simulink model "DrishtiSetu_Screening"  (R2026a)
settings: Solver=FixedStepDiscrete  StopTime=0  FixedStep=1
undefined symbols (not defined in the file or in its folder): sim_adherence, sim_camp_days, sim_devices, sim_dm_prev, sim_pop
settings Model: Creator=itsam  LastModifiedBy=itsam

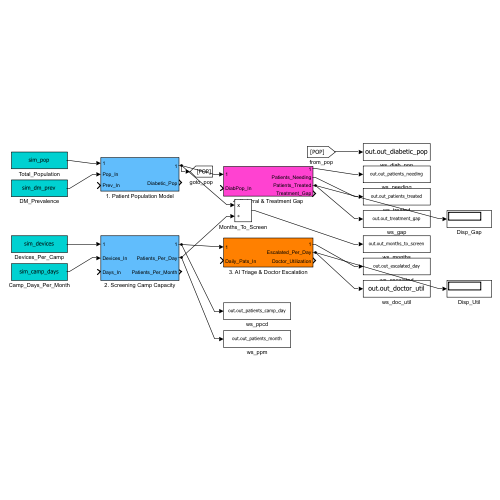
[thumbnail: Simulink's stored preview of the top-level diagram]
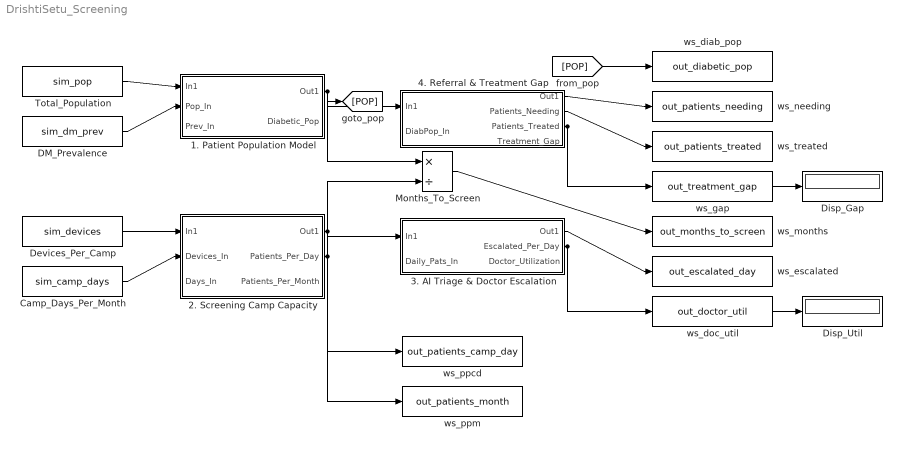
== system DrishtiSetu_Screening ==
  1. Patient Population Model : Subsystem
  2. Screening Camp Capacity : Subsystem
  3. AI Triage & Doctor Escalation : Subsystem
  4. Referral & Treatment Gap : Subsystem
  Camp_Days_Per_Month : Constant  Value=sim_camp_days
  DM_Prevalence : Constant  Value=sim_dm_prev
  Devices_Per_Camp : Constant  Value=sim_devices
  Disp_Gap : Display
  Disp_Util : Display
  Months_To_Screen : Product  Inputs=*/
  Total_Population : Constant  Value=sim_pop
  ws_diab_pop : ToWorkspace  VariableName=out_diabetic_pop  SaveFormat=Timeseries  SampleTime=-1
  ws_doc_util : ToWorkspace  VariableName=out_doctor_util  SaveFormat=Timeseries  SampleTime=-1
  ws_escalated : ToWorkspace  VariableName=out_escalated_day  SaveFormat=Timeseries  SampleTime=-1
  ws_gap : ToWorkspace  VariableName=out_treatment_gap  SaveFormat=Timeseries  SampleTime=-1
  ws_months : ToWorkspace  VariableName=out_months_to_screen  SaveFormat=Timeseries  SampleTime=-1
  ws_needing : ToWorkspace  VariableName=out_patients_needing  SaveFormat=Timeseries  SampleTime=-1
  ws_ppcd : ToWorkspace  VariableName=out_patients_camp_day  SaveFormat=Timeseries  SampleTime=-1
  ws_ppm : ToWorkspace  VariableName=out_patients_month  SaveFormat=Timeseries  SampleTime=-1
  ws_treated : ToWorkspace  VariableName=out_patients_treated  SaveFormat=Timeseries  SampleTime=-1
  wires:
  Total_Population/1 -> 1. Patient Population Model/1(In1)
  DM_Prevalence/1 -> 1. Patient Population Model/2(Pop_In)
  Devices_Per_Camp/1 -> 2. Screening Camp Capacity/1(In1)
  Camp_Days_Per_Month/1 -> 2. Screening Camp Capacity/2(Devices_In)
  2. Screening Camp Capacity/1(Out1) -> 3. AI Triage & Doctor Escalation/1(In1), ws_ppcd/1
  1. Patient Population Model/1(Out1) -> 4. Referral & Treatment Gap/1(In1), Months_To_Screen/1, [POP]
  2. Screening Camp Capacity/2(Patients_Per_Day) -> Months_To_Screen/2, ws_ppm/1
  [POP] -> ws_diab_pop/1
  4. Referral & Treatment Gap/1(Out1) -> ws_needing/1
  4. Referral & Treatment Gap/2(Patients_Needing) -> ws_treated/1
  4. Referral & Treatment Gap/3(Patients_Treated) -> ws_gap/1, Disp_Gap/1
  Months_To_Screen/1 -> ws_months/1
  3. AI Triage & Doctor Escalation/1(Out1) -> ws_escalated/1
  3. AI Triage & Doctor Escalation/2(Escalated_Per_Day) -> ws_doc_util/1, Disp_Util/1

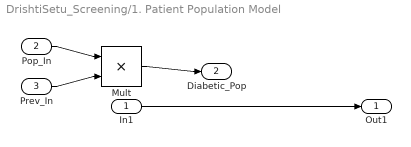
== system DrishtiSetu_Screening/1. Patient Population Model ==
  In1 : Inport
  Pop_In : Inport  Port=2
  Prev_In : Inport  Port=3
  Mult : Product
  Out1 : Outport
  Diabetic_Pop : Outport  Port=2
  wires:
  In1/1 -> Out1/1
  Pop_In/1 -> Mult/1
  Prev_In/1 -> Mult/2
  Mult/1 -> Diabetic_Pop/1

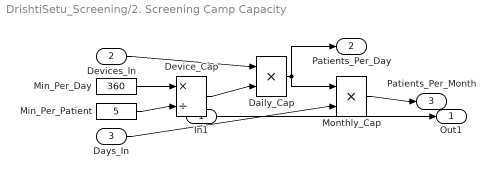
== system DrishtiSetu_Screening/2. Screening Camp Capacity ==
  In1 : Inport
  Devices_In : Inport  Port=2
  Days_In : Inport  Port=3
  Daily_Cap : Product
  Device_Cap : Product  Inputs=*/
  Min_Per_Day : Constant  Value=360
  Min_Per_Patient : Constant  Value=5
  Monthly_Cap : Product
  Out1 : Outport
  Patients_Per_Day : Outport  Port=2
  Patients_Per_Month : Outport  Port=3
  wires:
  In1/1 -> Out1/1
  Min_Per_Day/1 -> Device_Cap/1
  Min_Per_Patient/1 -> Device_Cap/2
  Devices_In/1 -> Daily_Cap/1
  Device_Cap/1 -> Daily_Cap/2
  Daily_Cap/1 -> Monthly_Cap/1, Patients_Per_Day/1
  Days_In/1 -> Monthly_Cap/2
  Monthly_Cap/1 -> Patients_Per_Month/1

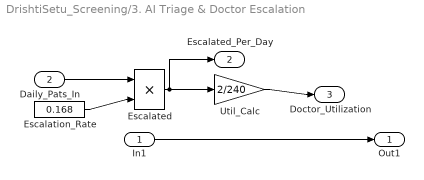
== system DrishtiSetu_Screening/3. AI Triage & Doctor Escalation ==
  In1 : Inport
  Daily_Pats_In : Inport  Port=2
  Escalated : Product
  Escalation_Rate : Constant  Value=0.168
  Util_Calc : Gain  Gain=2/240
  Out1 : Outport
  Escalated_Per_Day : Outport  Port=2
  Doctor_Utilization : Outport  Port=3
  wires:
  In1/1 -> Out1/1
  Daily_Pats_In/1 -> Escalated/1
  Escalation_Rate/1 -> Escalated/2
  Escalated/1 -> Util_Calc/1, Escalated_Per_Day/1
  Util_Calc/1 -> Doctor_Utilization/1

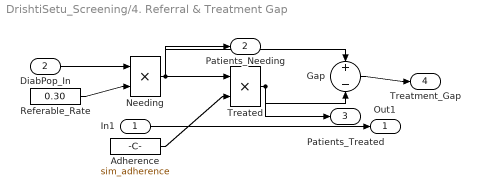
== system DrishtiSetu_Screening/4. Referral & Treatment Gap ==
  In1 : Inport
  DiabPop_In : Inport  Port=2
  Adherence : Constant  Value=sim_adherence
  Gap : Sum  Inputs=+-
  Needing : Product
  Referable_Rate : Constant  Value=0.30
  Treated : Product
  Out1 : Outport
  Patients_Needing : Outport  Port=2
  Patients_Treated : Outport  Port=3
  Treatment_Gap : Outport  Port=4
  wires:
  In1/1 -> Out1/1
  DiabPop_In/1 -> Needing/1
  Referable_Rate/1 -> Needing/2
  Needing/1 -> Patients_Needing/1, Treated/1, Gap/1
  Adherence/1 -> Treated/2
  Treated/1 -> Patients_Treated/1, Gap/2
  Gap/1 -> Treatment_Gap/1
